simulink model "Malhaaberta"  (R2023a)
settings: Solver=ode45  StartTime=0.0  StopTime=SampleTime  RelTol=1e-3  EnableMultiTasking=on
values from neighbouring files (symbols this model uses):
  b = 0.9    [setup.m]
  d = 0.5    [setup.m]
  g = 9.8    [setup.m]
  l = 1.5    [setup.m]
  M = 44    [setup.m]
  m = 3    [setup.m]
settings Model: Creator=05630646761  LastModifiedBy=pedro
settings SolverCC: AlgebraicLoopSolver=TrustRegion
settings DataIOCC: LimitDataPoints=on  SaveFormat=Array  ReturnWorkspaceOutputs=off
settings OptimizationCC: LifeSpan=inf
settings DebuggingCC: UnderspecifiedInitializationDetection=Classic  MergeDetectMultiDrivingBlocksExec=none  SolverPrmCheckMsg=warning  UnconnectedInputMsg=warning  UnconnectedOutputMsg=warning  UnconnectedLineMsg=warning  StateNameClashWarn=warning  SFUnexpectedBacktrackingDiag=warning  SFNoUnconditionalDefaultTransitionDiag=warning  SFExecutionAtInitializationDiag=none  ArithmeticOperatorsInVariantConditions=warning
settings HardwareCC: ProdBitPerPointer=32  ProdBitPerSizeT=32  ProdBitPerPtrDiffT=32  ProdLargestAtomicFloat=None  ProdIntDivRoundTo=Undefined  ProdEndianess=Unspecified  ProdWordSize=32  ProdHWDeviceType=32-bit Generic
settings ModelReferenceCC: PropagateSignalLabelsOutOfModel=off
settings SFSimCC: SimUseLocalCustomCode=off  CustomCodeUndefinedFunction=UseInterfaceOnly
settings RTWCC: RTWUseLocalCustomCode=off
settings CodeAppCC: StateflowObjectComments=on
settings GRTTargetCC: TargetLangStandard=C89/C90 (ANSI)
settings ConfigComp: CovMetricSettings=dw  CovSaveCumulativeToWorkspaceVar=on  CovSaveSingleToWorkspaceVar=on  CovExternalEMLEnable=off

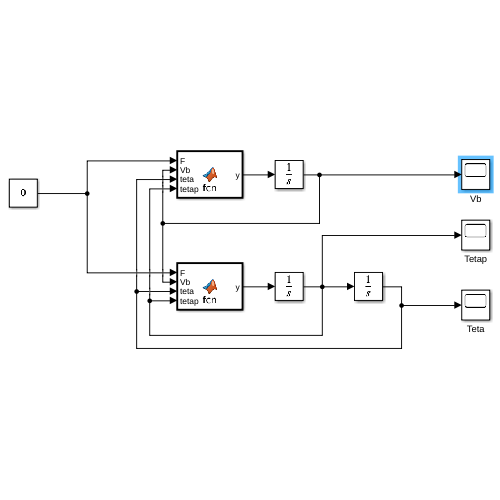
[thumbnail: Simulink's stored preview of the top-level diagram]
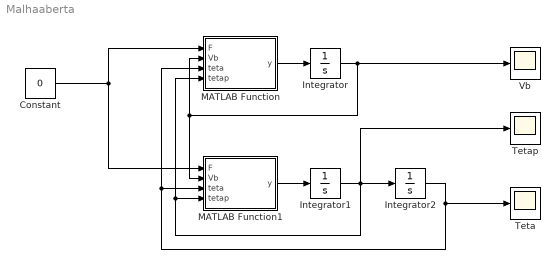
== system Malhaaberta ==
  Constant : Constant  Value=0
  Integrator : Integrator
  Integrator1 : Integrator
  Integrator2 : Integrator  InitialCondition=0.1
  MATLAB Function : MATLAB Function  TreatAsAtomicUnit=on
  MATLAB Function1 : MATLAB Function  TreatAsAtomicUnit=on
  Teta : Scope
  Tetap : Scope
  Vb : Scope
  wires:
  MATLAB Function/1(y) -> Integrator/1
  Integrator/1 -> Vb/1, MATLAB Function/2(Vb), MATLAB Function1/2(Vb)
  MATLAB Function1/1(y) -> Integrator1/1
  Integrator2/1 -> Teta/1, MATLAB Function1/3(teta), MATLAB Function/3(teta)
  Integrator1/1 -> Tetap/1, Integrator2/1, MATLAB Function1/4(tetap), MATLAB Function/4(tetap)
  Constant/1 -> MATLAB Function1/1(F), MATLAB Function/1(F)

== matlab function Malhaaberta/MATLAB Function1 ==
  data: F input; y output; Vb input; M parameter; m parameter; l parameter; teta input; tetap input; g parameter; d parameter; b parameter
function y = fcn(F, Vb,M, m, l, teta,tetap, g,d, b)


y = ( (M + m)*l*g*sin(teta) - ((M+m)/m)*b*tetap + l*cos(teta)*( F - d*Vb - m*l*sin(teta)*(tetap^2) )   )/( (l^2)*(M + m*((sin(teta))^2)) );

== matlab function Malhaaberta/MATLAB Function ==
  data: F input; y output; Vb input; M parameter; m parameter; l parameter; teta input; tetap input; g parameter; d parameter; b parameter
function y = fcn(F, Vb,M, m, l, teta,tetap, g, d, b)


y = ( F - d*Vb - m*l*sin(teta)*(tetap^2) + cos(teta)*sin(teta)*m*g - (cos(teta)/l)*b*tetap)/( M + m*(((sin(teta))^2)) );
